simulink model "C_Rate"  (R2024b)
settings: Solver=ode3  StartTime=0.0  StopTime=60  FixedStep=1e-5  RelTol=1e-3
undefined symbols (not defined in the file): Ion, Lithium
libraries: spsBatteryLib x8, spsSeriesRLCBranchLib x3, spsCurrentMeasurementLib x1, spsGroundLib x1, spsSeriesRLCLoadLib x1, spsVoltageMeasurementLib x1, sps_lib x1
settings Model: Creator=balaj  LastModifiedBy=balaj
settings SolverCC: ZeroCrossControl=DisableAll

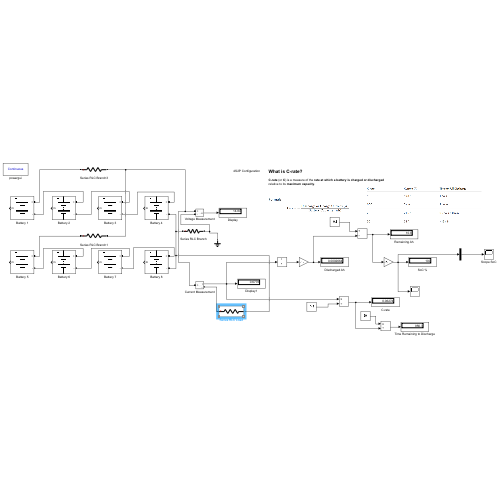
[thumbnail: Simulink's stored preview of the top-level diagram]
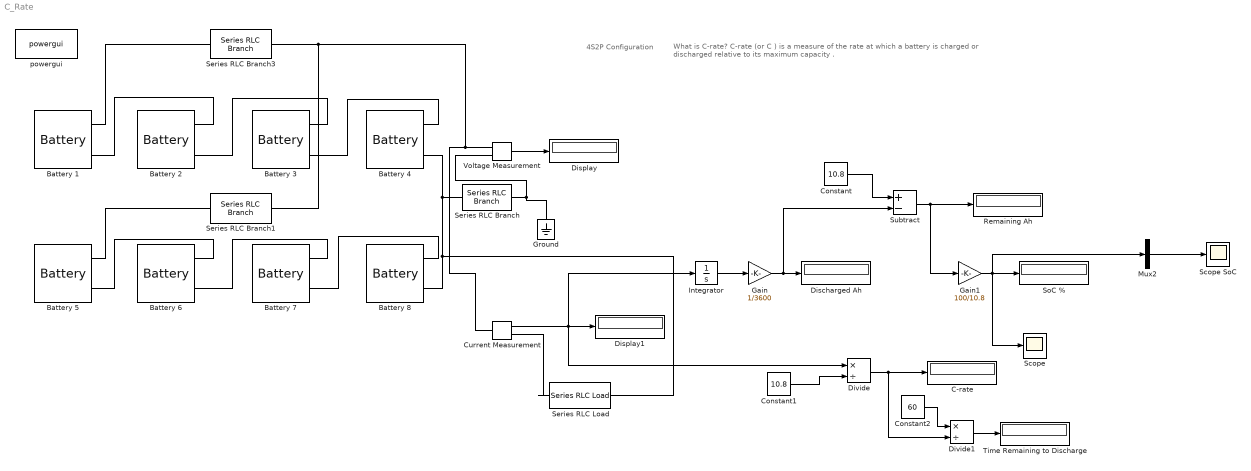
== system C_Rate ==
  note: What is C-rate?
      | C-rate (or C ) is a measure of the rate at which a battery is charged or discharged relative to its maximum capacity .
  note: 4S2P Configuration
  Battery {1..8} (8 alike) : spsBatteryLib/Battery  BatType=Lithium-Ion  NomV=3.2  NomQ=5.4  SOC=100  Batt_Tr=30  PresetModel=off  MaxQ=5.4  MinV=2.4  FullV=3.7  Dis_rate=2.3478  R=0.0059259  Normal_OP=4.8835  expZone="[3.4572      0.2653]"
  C-rate : Display
  Constant : Constant  Value=10.8
  Constant1 : Constant  Value=10.8
  Constant2 : Constant  Value=60
  Current Measurement : spsCurrentMeasurementLib/Current Measurement  PhasorSimulation=off  OutputType=Complex  PSBequivalent=0
  Discharged Ah : Display
  Display : Display
  Display1 : Display
  Divide : Product  Inputs=*/
  Divide1 : Product  Inputs=*/
  Gain : Gain  Gain=1/3600
  Gain1 : Gain  Gain=100/10.8
  Ground : spsGroundLib/Ground  LConnTagsString=a
  Integrator : Integrator
  Mux2 : Mux  Inputs=1
  Remaining Ah : Display
  Scope : Scope
  Scope SoC : Scope
  Series RLC Branch : spsSeriesRLCBranchLib/Series RLC Branch  LConnTagsString=__new0  RConnTagsString=__new0  BranchType=R  Resistance=0.01  Inductance=1e-3  SetiL0=off  InitialCurrent=0  Capacitance=1e-6  Setx0=off  InitialVoltage=0  Measurements=None
  Series RLC Branch1 : spsSeriesRLCBranchLib/Series RLC Branch  LConnTagsString=__new0  RConnTagsString=__new0  BranchType=R  Resistance=0.01  Inductance=1e-3  SetiL0=off  InitialCurrent=0  Capacitance=1e-6  Setx0=off  InitialVoltage=0  Measurements=None
  Series RLC Branch3 : spsSeriesRLCBranchLib/Series RLC Branch  LConnTagsString=__new0  RConnTagsString=__new0  BranchType=R  Resistance=0.01  Inductance=1e-3  SetiL0=off  InitialCurrent=0  Capacitance=1e-6  Setx0=off  InitialVoltage=0  Measurements=None
  Series RLC Load : spsSeriesRLCLoadLib/Series RLC Load  LConnTagsString=a  RConnTagsString=__new0  NominalVoltage=14.8  NominalFrequency=50  ActivePower=1  InductivePower=0  CapacitivePower=0  Setx0=off  InitialVoltage=0  SetiL0=off  InitialCurrent=0  Measurements=None  LoadType=constant Z
  SoC % : Display
  Subtract : Sum  Inputs=+-
  Time Remaining to Discharge : Display
  Voltage Measurement : spsVoltageMeasurementLib/Voltage Measurement  PhasorSimulation=off  OutputType=Complex  PSBequivalent=0
  powergui : sps_lib/powergui  Priority=1  SimulationMode=Continuous  SampleTime=50e-6  frequency=60  Iterations=50  frequencyindice=0  Pbase=100e6  ErrMax=1e-4  UnitsV=kV  UnitsW=MW  buscounter=0  FunctionMessages=off  echomessages=off  EnableUseOfTLC=off  CurrentSourceSwitches=off  DisableSnubberDevices=off  DisableRonSwitches=off  DisableVfSwitches=off  DisplayEquations=off  AutomaticDiscreteSolvers=off  SolverType=Tustin/Backward Euler (TBE)  Interpol=off  ExternalGateDelay=off  methode=off  Ts=100  x0status=blocks  SPID=on  SwTol=0  HookPort=off  NonlinearTolerance=1e-4  nMaxIteration=100  ContinueOnMaxIteration=off  RestoreLinks=warning  ResistiveCurrentMeasurement=off  Frange=[0:2:500]  Ylog=off  Xlog=on  ShowGrid=off  save=off  variable=ZData  structure=0  ZoomFFT=off  StartTime=0.0  cycles=1  DisplayStyle=1  fundamental=60  FreqAxis=off  MaxFrequency=1000  frequencyindicesteady=1  RmsSteady=1  display=off
  wires:
  Voltage Measurement/1 -> Display/1
  Current Measurement/1 -> Divide/1, Display1/1, Integrator/1
  Integrator/1 -> Gain/1
  Gain/1 -> Subtract/2, Discharged Ah/1
  Constant/1 -> Subtract/1
  Subtract/1 -> Gain1/1, Remaining Ah/1
  Gain1/1 -> Scope/1, Mux2/1, SoC %/1
  Mux2/1 -> Scope SoC/1
  Constant1/1 -> Divide/2
  Divide/1 -> Divide1/2, C-rate/1
  Constant2/1 -> Divide1/1
  Divide1/1 -> Time Remaining to Discharge/1
  connections:
  Battery 1/LConn2 -- Battery 2/LConn1
  Battery 2/LConn2 -- Battery 3/LConn1
  Battery 3/LConn2 -- Battery 4/LConn1
  Battery 5/LConn2 -- Battery 6/LConn1
  Battery 6/LConn2 -- Battery 7/LConn1
  Battery 7/LConn2 -- Battery 8/LConn1
  Battery 4/LConn2 -- Series RLC Load/RConn1 -- Battery 8/LConn2 -- Series RLC Branch/LConn1
  Series RLC Branch/RConn1 -- Ground/LConn1 -- Voltage Measurement/LConn2
  Series RLC Branch1/LConn1 -- Battery 5/LConn1
  Battery 1/LConn1 -- Series RLC Branch3/LConn1
  Series RLC Branch1/RConn1 -- Current Measurement/LConn1 -- Voltage Measurement/LConn1 -- Series RLC Branch3/RConn1
  Series RLC Load/LConn1 -- Current Measurement/RConn1
